simulink model "nn"  (R2024b)
settings: Solver=VariableStepAuto  StartTime=0.0  StopTime=10.0  RelTol=1e-3
libraries: neural x122
(part 1 of 5)
settings Model: Creator=wcheng2014  LastModifiedBy=wcheng2014

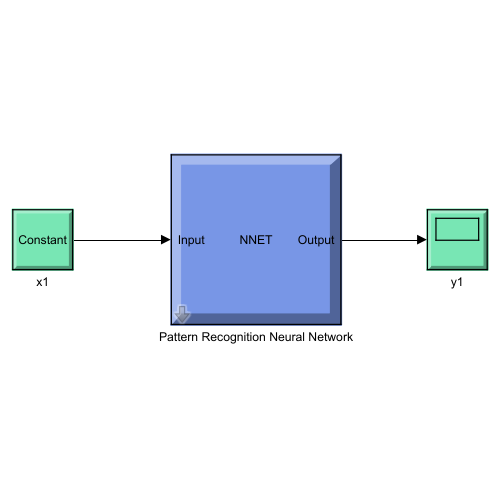
[thumbnail: Simulink's stored preview of the top-level diagram]
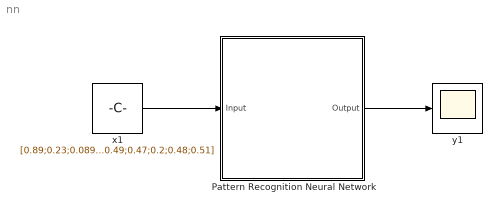
== system nn ==
  Pattern Recognition Neural Network : Subsystem
      mask help: Pattern Recognition Neural Network
      mask Display: e = 0.06;c1 = [120 150 230]/255;c2 = ([120 150 230]+0)/383;c3 = ([120 150 230]+128)/383;patch([0 1 1 0],[0 0 1 1],c1);patch([0 1 1 1-e 1-e 0+e],[0 0 1 1-e 0+e 0+e],c2);patch([0 0 1 1-e 0+e 0+e],[0 1 1 1-e 1-e 0+e],c3);plot([0 1 1 0 0],[0 0 1 1 0]);fprintf('NNET');port_label('input',1,' Input');port_label('output',1,'Output ');
  x1 : Constant  Value=[0.89;0.23;0.089;0.31;0.097;0.39;0.14;0.61;0.89;0.45;0.5;0.47;0.2;0.95;0.26;0.56;0.64;0.88;0.94;0.49;0.47;0.2;0.48;0.51]  SampleTime=1
      mask Display: e = 0.06;c1 = [120 230 180]/255;c2 = ([120 230 180]+0)/(256+128);c3 = ([120 230 180]+128)/(256+128);patch([0 1 1 0],[0 0 1 1],c1);patch([0 1 1 1-e 1-e 0+e],[0 0 1 1-e 0+e 0+e],c2);patch([0 0 1 1-e 0+e 0+e],[0 1 1 1-e 1-e 0+e],c3);plot([0 1 1 0 0],[0 0 1 1 0]);disp('Constant');
  y1 : Scope
      mask Display: e = 0.06;c1 = [120 230 180]/255;c2 = ([120 230 180]+0)/(256+128);c3 = ([120 230 180]+128)/(256+128);patch([0 1 1 0],[0 0 1 1],c1);patch([0 1 1 1-e 1-e 0+e],[0 0 1 1-e 0+e 0+e],c2);patch([0 0 1 1-e 0+e 0+e],[0 1 1 1-e 1-e 0+e],c3);plot([0 1 1 0 0],[0 0 1 1 0]);plot([0.15 0.85 0.85 0.15 0.15],[0.5 0.5 0.85 0.85 0.5]);
  wires:
  x1/1 -> Pattern Recognition Neural Network/1(Input)
  Pattern Recognition Neural Network/1(Output) -> y1/1

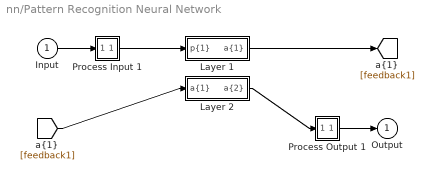
== system nn/Pattern Recognition Neural Network ==
  Input : Inport  PortDimensions=24
      mask Display: e = 0.06;c1 = [120 230 180]/255;c2 = ([120 230 180]+0)/(256+128);c3 = ([120 230 180]+128)/(256+128);patch([0 1 1 0],[0 0 1 1],c1);patch([0 1 1 1-e 1-e 0+e],[0 0 1 1-e 0+e 0+e],c2);patch([0 0 1 1-e 0+e 0+e],[0 1 1 1-e 1-e 0+e],c3);plot([0 1 1 0 0],[0 0 1 1 0]);
  Layer 1 : Subsystem
      mask Display: e = 0.06;c1 = [120 150 230]/255;c2 = ([120 150 230]+0)/383;c3 = ([120 150 230]+128)/383;patch([0 1 1 0],[0 0 1 1],c1);patch([0 1 1 1-e 1-e 0+e],[0 0 1 1-e 0+e 0+e],c2);patch([0 0 1 1-e 0+e 0+e],[0 1 1 1-e 1-e 0+e],c3);plot([0 1 1 0 0],[0 0 1 1 0]);
  Layer 2 : Subsystem
      mask Display: e = 0.06;c1 = [120 150 230]/255;c2 = ([120 150 230]+0)/383;c3 = ([120 150 230]+128)/383;patch([0 1 1 0],[0 0 1 1],c1);patch([0 1 1 1-e 1-e 0+e],[0 0 1 1-e 0+e 0+e],c2);patch([0 0 1 1-e 0+e 0+e],[0 1 1 1-e 1-e 0+e],c3);plot([0 1 1 0 0],[0 0 1 1 0]);
  Process Input 1 : Subsystem
      mask Display: e = 0.06;c1 = [120 150 230]/255;c2 = ([120 150 230]+0)/383;c3 = ([120 150 230]+128)/383;patch([0 1 1 0],[0 0 1 1],c1);patch([0 1 1 1-e 1-e 0+e],[0 0 1 1-e 0+e 0+e],c2);patch([0 0 1 1-e 0+e 0+e],[0 1 1 1-e 1-e 0+e],c3);plot([0 1 1 0 0],[0 0 1 1 0]);
  Process Output 1 : Subsystem
      mask Display: e = 0.06;c1 = [120 150 230]/255;c2 = ([120 150 230]+0)/383;c3 = ([120 150 230]+128)/383;patch([0 1 1 0],[0 0 1 1],c1);patch([0 1 1 1-e 1-e 0+e],[0 0 1 1-e 0+e 0+e],c2);patch([0 0 1 1-e 0+e 0+e],[0 1 1 1-e 1-e 0+e],c3);plot([0 1 1 0 0],[0 0 1 1 0]);
  Output : Outport  InitialOutput=[0;0;0;0;0;0;0;0;0;0;0;0;0;0;0;0;0;0;0]
      mask Display: e = 0.06;c1 = [120 230 180]/255;c2 = ([120 230 180]+0)/(256+128);c3 = ([120 230 180]+128)/(256+128);patch([0 1 1 0],[0 0 1 1],c1);patch([0 1 1 1-e 1-e 0+e],[0 0 1 1-e 0+e 0+e],c2);patch([0 0 1 1-e 0+e 0+e],[0 1 1 1-e 1-e 0+e],c3);plot([0 1 1 0 0],[0 0 1 1 0]);
  wires:
  Input/1 -> Process Input 1/1(x)
  Process Output 1/1(y) -> Output/1
  Process Input 1/1(p) -> Layer 1/1("p{1}")
  Layer 1/1("a{1}") -> [feedback1]
  [feedback1] -> Layer 2/1("a{1} ")
  Layer 2/1("a{2}") -> Process Output 1/1(a)

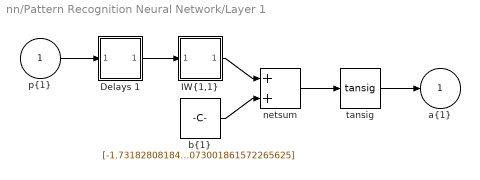
== system nn/Pattern Recognition Neural Network/Layer 1 ==
  "p{1}" : Inport  PortDimensions=24
      mask Display: e = 0.06;c1 = [120 230 180]/255;c2 = ([120 230 180]+0)/(256+128);c3 = ([120 230 180]+128)/(256+128);patch([0 1 1 0],[0 0 1 1],c1);patch([0 1 1 1-e 1-e 0+e],[0 0 1 1-e 0+e 0+e],c2);patch([0 0 1 1-e 0+e 0+e],[0 1 1 1-e 1-e 0+e],c3);plot([0 1 1 0 0],[0 0 1 1 0]);
  Delays 1 : Subsystem
      mask Display: e = 0.06;c1 = [120 150 230]/255;c2 = ([120 150 230]+0)/383;c3 = ([120 150 230]+128)/383;patch([0 1 1 0],[0 0 1 1],c1);patch([0 1 1 1-e 1-e 0+e],[0 0 1 1-e 0+e 0+e],c2);patch([0 0 1 1-e 0+e 0+e],[0 1 1 1-e 1-e 0+e],c3);plot([0 1 1 0 0],[0 0 1 1 0]);disp('0');
  "IW{1,1}" : Subsystem
      mask Display: e = 0.06;c1 = [120 150 230]/255;c2 = ([120 150 230]+0)/383;c3 = ([120 150 230]+128)/383;patch([0 1 1 0],[0 0 1 1],c1);patch([0 1 1 1-e 1-e 0+e],[0 0 1 1-e 0+e 0+e],c2);patch([0 0 1 1-e 0+e 0+e],[0 1 1 1-e 1-e 0+e],c3);plot([0 1 1 0 0],[0 0 1 1 0]);disp('W');
  "b{1}" : Constant  Value=[-1.7318280818438103185741283596144057810306549072265625;-1.8894955860517779200336008216254413127899169921875;-1.883601561975761118361560875200666487216949462890625;1.297914296781323972851396320038475096225738525390625;1.677994924977186830261643990525044500827789306640625;1.6859882770272276442113934535882435739040374755859375;-1.5219376217309024124091365592903457581996917724609375;-1.3771115518127394761194182137842290103435516357421875;1.5190144572738695227798189080203883349895477294921875;1.7054716163176510956844822430866770446300506591796875;-1.403204461630382038350717266439460217952728271484375;1.3510711629585088200400377900223247706890106201171875;1.2882379387234272893891784406150691211223602294921875;1.027581673753412250249539283686317503452301025390625;-1.4689946955028896358186329962336458265781402587890625;-1.54831643517333272797031895606778562068939208984375;1.2318122216712896754842176960664801299571990966796875;-1.011976579315719160234721130109392106533050537109375;-1.2911269821805995139385458969627507030963897705078125;-1.6279110269177372583015994678135029971599578857421875;1.2074797993936015050309151774854399263858795166015625;-0.66327856053885592135799242896609939634799957275390625;-0.8350840552610232503383258517715148627758026123046875;0.73931517760920251181033790999208576977252960205078125;-1.148671497822288500856302562169730663299560546875;-1.0798007484762657259835805234615691006183624267578125;1.1684022346796982816385934711433947086334228515625;-1.0225826702826263936429995737853460013866424560546875;0.55256932693761495745121692380052991211414337158203125;0.001919523026375129746978753786379456869326531887054443359375;-0.52738977712046664070300039384164847433567047119140625;-0.85521358685274495581296605450916104018688201904296875;0.61862792626946283558453387740883044898509979248046875;-0.310695263153003942147023508368874900043010711669921875;0.803025143184609380142546797287650406360626220703125;0.2114801559340895587002506772478227503597736358642578125;-0.26370804480799581170913370442576706409454345703125;-0.7810372740686679637889255900518037378787994384765625;0.70268290336174865640117559451027773320674896240234375;0.57980506267781262152993804193101823329925537109375;0.477677937198980606670062343255267478525638580322265625;0.6306812405713078106828106683678925037384033203125;-0.4363250598704571103780835983343422412872314453125;0.25694629027165871715254752416512928903102874755859375;0.047143299392337086051174566136978683061897754669189453125;0.39043633281427514436501269301516003906726837158203125;-0.29527247698673597664509316018666140735149383544921875;-0.17818401746455470036067936234758235514163970947265625;-0.17348881198850640839026482353801839053630828857421875;-0.334985869906453459510231596141238696873188018798828125;0.29380531432906431543727876487537287175655364990234375;0.387762785015334066063275031410739757120609283447265625;0.235456742655576090061941840758663602173328399658203125;0.495069807714873688642143179095000959932804107666015625;0.73594194078101515810175214937771670520305633544921875;0.353487592149325069446064162548282183706760406494140625;-0.452364954469045399410020991126657463610172271728515625;0.3200648042724429931382701397524215281009674072265625;-0.65329653331767401081009438712499104440212249755859375;0.12352674901778253058193257629682193510234355926513671875;-0.385135835097819401173779851887957192957401275634765625;-0.187054791956881627523756606024107895791530609130859375;-0.6699226878429682674465084346593357622623443603515625;-1.054497740719244180951363887288607656955718994140625;0.74791300133695448604242983492440544068813323974609375;1.02616003072412187435702435323037207126617431640625;-0.285116728970916499807941590916016139090061187744140625;-0.8792947828777750718387551387422718107700347900390625;0.39335580572510508989836353066493757069110870361328125;1.024466491904188369943540237727575004100799560546875;-0.904698316349697773119942212360911071300506591796875 ...(+1603 chars)]
      mask Display: e = 0.06;c1 = [120 150 230]/255;c2 = ([120 150 230]+0)/383;c3 = ([120 150 230]+128)/383;patch([0 1 1 0],[0 0 1 1],c1);patch([0 1 1 1-e 1-e 0+e],[0 0 1 1-e 0+e 0+e],c2);patch([0 0 1 1-e 0+e 0+e],[0 1 1 1-e 1-e 0+e],c3);plot([0 1 1 0 0],[0 0 1 1 0]);disp('b');
  netsum : Sum  Inputs=2  InputSameDT=on  SaturateOnIntegerOverflow=on  OutDataTypeStr=Inherit: Same as first input
      mask Display: e = 0.06;c1 = [120 150 230]/255;c2 = ([120 150 230]+0)/383;c3 = ([120 150 230]+128)/383;patch([0 1 1 0],[0 0 1 1],c1);patch([0 1 1 1-e 1-e 0+e],[0 0 1 1-e 0+e 0+e],c2);patch([0 0 1 1-e 0+e 0+e],[0 1 1 1-e 1-e 0+e],c3);plot([0 1 1 0 0],[0 0 1 1 0]);disp('+');
  tansig : neural/Transfer Functions/tansig
  "a{1}" : Outport  InitialOutput=[0;0;0;0;0;0;0;0;0;0;0;0;0;0;0;0;0;0;0;0;0;0;0;0;0;0;0;0;0;0;0;0;0;0;0;0;0;0;0;0;0;0;0;0;0;0;0;0;0;0;0;0;0;0;0;0;0;0;0;0;0;0;0;0;0;0;0;0;0;0;0;0;0;0;0;0;0;0;0;0;0;0;0;0;0;0;0;0;0;0;0;0;0;0;0;0;0;0;0;0]
      mask Display: e = 0.06;c1 = [120 230 180]/255;c2 = ([120 230 180]+0)/(256+128);c3 = ([120 230 180]+128)/(256+128);patch([0 1 1 0],[0 0 1 1],c1);patch([0 1 1 1-e 1-e 0+e],[0 0 1 1-e 0+e 0+e],c2);patch([0 0 1 1-e 0+e 0+e],[0 1 1 1-e 1-e 0+e],c3);plot([0 1 1 0 0],[0 0 1 1 0]);
  wires:
  "p{1}"/1 -> Delays 1/1("p{1}")
  Delays 1/1("pd{1,1}") -> "IW{1,1}"/1("pd{1,1}")
  "IW{1,1}"/1("iz{1,1}") -> netsum/1
  "b{1}"/1 -> netsum/2
  netsum/1 -> tansig/1
  tansig/1 -> "a{1}"/1

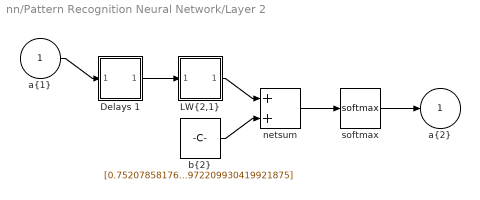
== system nn/Pattern Recognition Neural Network/Layer 2 ==
  "a{1} " : Inport  PortDimensions=100
      mask Display: e = 0.06;c1 = [120 230 180]/255;c2 = ([120 230 180]+0)/(256+128);c3 = ([120 230 180]+128)/(256+128);patch([0 1 1 0],[0 0 1 1],c1);patch([0 1 1 1-e 1-e 0+e],[0 0 1 1-e 0+e 0+e],c2);patch([0 0 1 1-e 0+e 0+e],[0 1 1 1-e 1-e 0+e],c3);plot([0 1 1 0 0],[0 0 1 1 0]);
  Delays 1 : Subsystem
      mask Display: e = 0.06;c1 = [120 150 230]/255;c2 = ([120 150 230]+0)/383;c3 = ([120 150 230]+128)/383;patch([0 1 1 0],[0 0 1 1],c1);patch([0 1 1 1-e 1-e 0+e],[0 0 1 1-e 0+e 0+e],c2);patch([0 0 1 1-e 0+e 0+e],[0 1 1 1-e 1-e 0+e],c3);plot([0 1 1 0 0],[0 0 1 1 0]);disp('0');
  "LW{2,1}" : Subsystem
      mask Display: e = 0.06;c1 = [120 150 230]/255;c2 = ([120 150 230]+0)/383;c3 = ([120 150 230]+128)/383;patch([0 1 1 0],[0 0 1 1],c1);patch([0 1 1 1-e 1-e 0+e],[0 0 1 1-e 0+e 0+e],c2);patch([0 0 1 1-e 0+e 0+e],[0 1 1 1-e 1-e 0+e],c3);plot([0 1 1 0 0],[0 0 1 1 0]);disp('W');
  "b{2}" : Constant  Value=[0.7520785817646882254194906636257655918598175048828125;0.71391572920923851430785589400329627096652984619140625;0.6945604420730118189197810352197848260402679443359375;-0.50055811124942606316068349769921042025089263916015625;-0.77692786430216209669907811985467560589313507080078125;0.015641384517091759531748351719215861521661281585693359375;0.485821131956972795951088528454420156776905059814453125;-0.94792672012345147170009340698015876114368438720703125;-0.16653488906920677070644387640641070902347564697265625;-0.51023059158994954476185057501425035297870635986328125;0.5908541035176517741689394824788905680179595947265625;-0.36682659034473708015156034889514558017253875732421875;-1.0709892922752308752620820087031461298465728759765625;-0.85856970819947975304131659868289716541767120361328125;-0.65000439077791904995962113389396108686923980712890625;0.9072072595770388492297797711216844618320465087890625;-0.0038011840110758984313810149302526042447425425052642822265625;0.63492717479604998676023797088419087231159210205078125;-0.1216193960094091586210396371825481764972209930419921875]
      mask Display: e = 0.06;c1 = [120 150 230]/255;c2 = ([120 150 230]+0)/383;c3 = ([120 150 230]+128)/383;patch([0 1 1 0],[0 0 1 1],c1);patch([0 1 1 1-e 1-e 0+e],[0 0 1 1-e 0+e 0+e],c2);patch([0 0 1 1-e 0+e 0+e],[0 1 1 1-e 1-e 0+e],c3);plot([0 1 1 0 0],[0 0 1 1 0]);disp('b');
  netsum : Sum  Inputs=2  InputSameDT=on  SaturateOnIntegerOverflow=on  OutDataTypeStr=Inherit: Same as first input
      mask Display: e = 0.06;c1 = [120 150 230]/255;c2 = ([120 150 230]+0)/383;c3 = ([120 150 230]+128)/383;patch([0 1 1 0],[0 0 1 1],c1);patch([0 1 1 1-e 1-e 0+e],[0 0 1 1-e 0+e 0+e],c2);patch([0 0 1 1-e 0+e 0+e],[0 1 1 1-e 1-e 0+e],c3);plot([0 1 1 0 0],[0 0 1 1 0]);disp('+');
  softmax : neural/Transfer Functions/softmax
  "a{2}" : Outport  InitialOutput=[0;0;0;0;0;0;0;0;0;0;0;0;0;0;0;0;0;0;0]
      mask Display: e = 0.06;c1 = [120 230 180]/255;c2 = ([120 230 180]+0)/(256+128);c3 = ([120 230 180]+128)/(256+128);patch([0 1 1 0],[0 0 1 1],c1);patch([0 1 1 1-e 1-e 0+e],[0 0 1 1-e 0+e 0+e],c2);patch([0 0 1 1-e 0+e 0+e],[0 1 1 1-e 1-e 0+e],c3);plot([0 1 1 0 0],[0 0 1 1 0]);
  wires:
  "a{1} "/1 -> Delays 1/1("p{2}")
  Delays 1/1("pd{2,1}") -> "LW{2,1}"/1("ad{2,1}")
  "LW{2,1}"/1("lz{2,1}") -> netsum/1
  "b{2}"/1 -> netsum/2
  netsum/1 -> softmax/1
  softmax/1 -> "a{2}"/1

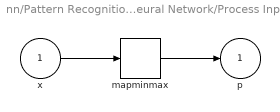
== system nn/Pattern Recognition Neural Network/Process Input 1 ==
  x : Inport  PortDimensions=24
      mask Display: e = 0.06;c1 = [120 230 180]/255;c2 = ([120 230 180]+0)/(256+128);c3 = ([120 230 180]+128)/(256+128);patch([0 1 1 0],[0 0 1 1],c1);patch([0 1 1 1-e 1-e 0+e],[0 0 1 1-e 0+e 0+e],c2);patch([0 0 1 1-e 0+e 0+e],[0 1 1 1-e 1-e 0+e],c3);plot([0 1 1 0 0],[0 0 1 1 0]);
  mapminmax : neural/Processing Functions/mapminmax  xmin=[-4.58529038245281128638453083113e-05;-0.000201141805104221305100509198382;-0.00426567193827276369688661361579;-0.000237777253548454581277837860398;-0.000302124233470646430532724480145;-0.000170828487644492099661874817684;-0.00438947468810502172686938138213;-0.000240426928764136960126052144915;-0.0036918438568669387223053490743;-0.00694340205276233746189973317087;-0.0012255717858442594092593935784;-0.00443299483310743980268853192683;-6.27443980936170930817752378061e-05;-0.000364964014374802303564138128422;-0.0019722402340520694963288406143;-0.00526332098432114037223072955385;-0.0026213409547284349798701441614;-0.00276425746896791224571643397212;-0.000510026570787580624255497241393;-0.00335199284059450874906360695604;-0.00415969258899906435544835403562;-0.00327300531995344812230541720055;-0.00197721111596038667812536004931;-0.00307281536089298867864272324368]  xmax=[0.0139064553203960272753647586796;0.015737716778017496466191005311;0.0119434492486112375786433403846;0.0136137130372100401132229308132;0.0102106167377793433104216092033;0.011662271042181870939202781301;0.00572056990158431588611165352631;0.00814735282962164575337737915106;0.00776714859349647568365071492735;0.00538260804221435407157514418941;0.00722011582307802157743026327807;0.00417593766836432678246637806296;0.00530125420928184709623565140646;0.00414630231089851974957127822563;0.00406636470585652887166361324489;0.00302482463683384494856909441296;0.000812733410832766622888811980374;0.000698867683294412955774532747455;0.00298852862990983680901990737766;0.00302429027532635785746606416069;0.00291193290581848174269907758571;0.00700753425606803759251306473743;0.00297790763760508170321372745093;0.00253836755213177056589302083012]  ymin=-1  ymax=1
  p : Outport  PortDimensions=24
      mask Display: e = 0.06;c1 = [120 230 180]/255;c2 = ([120 230 180]+0)/(256+128);c3 = ([120 230 180]+128)/(256+128);patch([0 1 1 0],[0 0 1 1],c1);patch([0 1 1 1-e 1-e 0+e],[0 0 1 1-e 0+e 0+e],c2);patch([0 0 1 1-e 0+e 0+e],[0 1 1 1-e 1-e 0+e],c3);plot([0 1 1 0 0],[0 0 1 1 0]);
  wires:
  x/1 -> mapminmax/1
  mapminmax/1 -> p/1

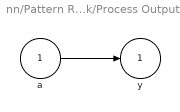
== system nn/Pattern Recognition Neural Network/Process Output 1 ==
  a : Inport  PortDimensions=19
      mask Display: e = 0.06;c1 = [120 230 180]/255;c2 = ([120 230 180]+0)/(256+128);c3 = ([120 230 180]+128)/(256+128);patch([0 1 1 0],[0 0 1 1],c1);patch([0 1 1 1-e 1-e 0+e],[0 0 1 1-e 0+e 0+e],c2);patch([0 0 1 1-e 0+e 0+e],[0 1 1 1-e 1-e 0+e],c3);plot([0 1 1 0 0],[0 0 1 1 0]);
  y : Outport  PortDimensions=19
      mask Display: e = 0.06;c1 = [120 230 180]/255;c2 = ([120 230 180]+0)/(256+128);c3 = ([120 230 180]+128)/(256+128);patch([0 1 1 0],[0 0 1 1],c1);patch([0 1 1 1-e 1-e 0+e],[0 0 1 1-e 0+e 0+e],c2);patch([0 0 1 1-e 0+e 0+e],[0 1 1 1-e 1-e 0+e],c3);plot([0 1 1 0 0],[0 0 1 1 0]);
  wires:
  a/1 -> y/1

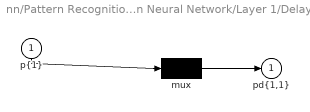
== system nn/Pattern Recognition Neural Network/Layer 1/Delays 1 ==
  "p{1}" : Inport  PortDimensions=24
      mask Display: e = 0.06;c1 = [120 230 180]/255;c2 = ([120 230 180]+0)/(256+128);c3 = ([120 230 180]+128)/(256+128);patch([0 1 1 0],[0 0 1 1],c1);patch([0 1 1 1-e 1-e 0+e],[0 0 1 1-e 0+e 0+e],c2);patch([0 0 1 1-e 0+e 0+e],[0 1 1 1-e 1-e 0+e],c3);plot([0 1 1 0 0],[0 0 1 1 0]);
  mux : Mux  Inputs=1
      mask Display: e = 0.06;c1 = [120 150 230]/255;c2 = ([120 150 230]+0)/383;c3 = ([120 150 230]+128)/383;patch([0 1 1 0],[0 0 1 1],c1);patch([0 1 1 1-e 1-e 0+e],[0 0 1 1-e 0+e 0+e],c2);patch([0 0 1 1-e 0+e 0+e],[0 1 1 1-e 1-e 0+e],c3);plot([0 1 1 0 0],[0 0 1 1 0]);disp('Mux')
  "pd{1,1}" : Outport
      mask Display: e = 0.06;c1 = [120 230 180]/255;c2 = ([120 230 180]+0)/(256+128);c3 = ([120 230 180]+128)/(256+128);patch([0 1 1 0],[0 0 1 1],c1);patch([0 1 1 1-e 1-e 0+e],[0 0 1 1-e 0+e 0+e],c2);patch([0 0 1 1-e 0+e 0+e],[0 1 1 1-e 1-e 0+e],c3);plot([0 1 1 0 0],[0 0 1 1 0]);
  wires:
  "p{1}"/1 -> mux/1
  mux/1 -> "pd{1,1}"/1
